simulink model "model_sim"  (R2016a)
settings: Solver=ode4  StartTime=0.0  StopTime=10.0  FixedStep=0.001  MaxStep=0.01  RelTol=1e-3
values from neighbouring files (symbols this model uses):
  lin = 1    [obiekt2.m]    (also in torque_x0.m; zad1.m = 10)
  p = 60    [zad1.m]
  Rn = 0.0185    [obiekt2.m]    (also in zad1.m)
libraries: simulink x2
settings Model: Creator=Maciek  LastModifiedBy=Maciek

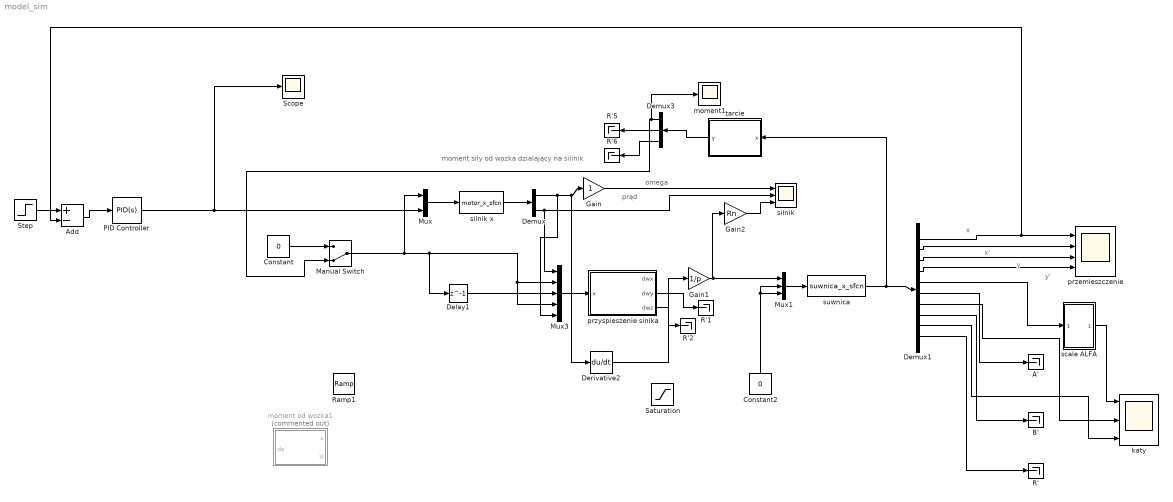
== system model_sim ==
  note: moment siły od wozka dzialający na silinik
  note: prąd
  note: omega
  note: y'
  note: y
  note: x'
  note: x
  A' : Terminator
  Add : Sum  Inputs=+-
  B' : Terminator
  Constant : Constant  Value=0
  Constant2 : Constant  Value=0
  Delay1 : Delay  DelayLength=1
  Demux : Demux  Outputs=2
  Demux1 : Demux  Outputs=10
  Demux3 : Demux  Outputs=3
  Derivative2 : Derivative
  Gain : Gain
  Gain1 : Gain  Gain=1/p
  Gain2 : Gain  Gain=Rn
  Manual Switch : ManualSwitch  CurrentSetting=0
  Mux : Mux  Inputs=2
  Mux1 : Mux  Inputs=3
  Mux3 : Mux  Inputs=5
  PID Controller : simulink/Continuous/PID Controller  Controller=PID  TimeDomain=Continuous-time  SampleTime=-1  IntegratorMethod=Forward Euler  FilterMethod=Forward Euler  Form=Parallel  UseFilter=on  ControllerParametersSource=internal  P=100  I=0.02  D=5  N=100  InitialConditionSource=internal  InitialConditionForIntegrator=0  InitialConditionForFilter=0  ExternalReset=none  LimitOutput=on  UpperSaturationLimit=20  LowerSaturationLimit=-20  LinearizeAsGain=on  AntiWindupMode=none  Kb=1  TrackingMode=off  Kt=1  PParamMin=[]  PParamMax=[]  IParamMin=[]  IParamMax=[]  DParamMin=[]  DParamMax=[]  NParamMin=[]  NParamMax=[]  KbParamMin=[]  KbParamMax=[]  KtParamMin=[]  KtParamMax=[]  POutMin=[]  POutMax=[]  IOutMin=[]  IOutMax=[]  DOutMin=[]  DOutMax=[]  NOutMin=[]  NOutMax=[]  KbOutMin=[]  KbOutMax=[]  KtOutMin=[]  KtOutMax=[]  IntegratorOutMin=[]  IntegratorOutMax=[]  FilterOutMin=[]  FilterOutMax=[]  SumOutMin=[]  SumOutMax=[]  SumI1OutMin=[]  SumI1OutMax=[]  SumI2OutMin=[]  SumI2OutMax=[]  SumI3OutMin=[]  SumI3OutMax=[]  SumDOutMin=[]  SumDOutMax=[]  SaturationOutMin=[]  SaturationOutMax=[]  IntegratorContinuousStateAttributes=''  IntegratorStateMustResolveToSignalObject=off  IntegratorRTWStateStorageClass=Auto  FilterContinuousStateAttributes=''  FilterStateMustResolveToSignalObject=off  FilterRTWStateStorageClass=Auto  DifferentiatorICPrevScaledInput=0  DifferentiatorOutMin=[]  DifferentiatorOutMax=[]
  R'{,1..2,5..6} (5 alike) : Terminator
  Ramp1 : simulink/Sources/Ramp  slope=0.5  start=0  X0=0
  Saturation : Saturate  UpperLimit=10  LowerLimit=-10
  Scope : Scope
  Step : Step  After=0.2  SampleTime=0
  katy : Scope  NumInputPorts=3
  moment od wozka1 : MATLAB Function  Commented=on  TreatAsAtomicUnit=on
  moment1 : Scope
  przemieszczenie : Scope  NumInputPorts=4
  przyspieszenie sinika : MATLAB Function  TreatAsAtomicUnit=on
  scale ALFA : Subsystem
  silnik : Scope  NumInputPorts=3
  silnik x : S-Function  FunctionName=motor_x_sfcn  SFunctionDeploymentMode=off  EnableBusSupport=off
  suwnica : S-Function  FunctionName=suwnica_x_sfcn  Parameters=x0  SFunctionDeploymentMode=off  EnableBusSupport=off
  tarcie : MATLAB Function  TreatAsAtomicUnit=on
  wires:
  Mux/1 -> silnik x/1
  silnik x/1 -> Demux/1
  Demux/1 -> Mux3/5, Derivative2/1, Gain/1
  Mux1/1 -> suwnica/1
  Constant2/1 -> Mux1/2, Mux1/3
  Demux1/10 -> R'/1
  Demux1/8 -> B'/1
  Demux1/7 -> katy/2
  Demux1/9 -> katy/3
  Demux1/6 -> A'/1
  Demux1/2 -> przemieszczenie/2
  Demux1/3 -> przemieszczenie/3
  Demux1/4 -> przemieszczenie/4
  Mux3/1 -> przyspieszenie sinika/1(x)
  przyspieszenie sinika/3(dwz) -> R'2/1
  przyspieszenie sinika/2(dwy) -> R'1/1
  suwnica/1 -> tarcie/1(x), Demux1/1
  Gain/1 -> silnik/1
  Demux/2 -> Mux3/1, silnik/2
  Delay1/1 -> Mux3/3
  Constant/1 -> Manual Switch/1
  Gain2/1 -> silnik/3
  tarcie/1(y) -> Demux3/1
  Demux3/2 -> R'5/1
  Demux3/3 -> R'6/1
  Demux3/1 -> moment1/1, Manual Switch/2
  Gain1/1 -> Mux1/1, Gain2/1
  Demux1/5 -> scale ALFA/1(In1)
  Demux1/1 -> Add/2, przemieszczenie/1
  scale ALFA/1(Out1) -> katy/1
  Manual Switch/1 -> Mux/1, Mux3/4, Mux3/2, Delay1/1
  PID Controller/1 -> Scope/1, Mux/2
  Add/1 -> PID Controller/1
  Step/1 -> Add/1
  Derivative2/1 -> Gain1/1

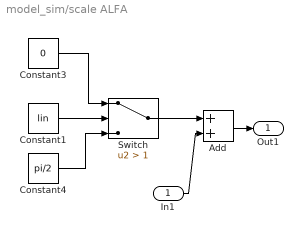
== system model_sim/scale ALFA ==
  In1 : Inport
  Add : Sum  Inputs=2
  Constant1 : Constant  Value=lin
  Constant3 : Constant  Value=0
  Constant4 : Constant  Value=pi/2
  Switch : Switch  Criteria=u2 > Threshold  Threshold=1
  Out1 : Outport
  wires:
  Add/1 -> Out1/1
  In1/1 -> Add/2
  Constant4/1 -> Switch/3
  Constant3/1 -> Switch/1
  Switch/1 -> Add/1
  Constant1/1 -> Switch/2

== matlab function model_sim/przyspieszenie sinika ==
  data: x input; dwx output; dwy output; dwz output
function [dwx, dwy, dwz] = angular_accel(x)

    %w = x(1); %predkosc katowa
    %temp = x(1);
    %ix = temp(2);
    wx = x(5);
    ix = x(1); % prad x
    iy = x(2); % prad x
    awx = x(3); %przysp x
    awy = x(4); %przys y
    
    xs = 1.5;   % szerokość suwnicy
    sy = 2.5;   % dł suwnicy
    mw = 1.155;%2.49;  % masa wózka
    ms = 2.2;%4.09;  % masa szyny
    mc = 1;     % masa ciężarka
    Rn = 0.0185;% promien bloków napedzajacych
    g = 9.81;
    p = 60;%przekladnia
    
    J = 1.1418*10^(-6);   %moment bezwladnisci
    tau_e = 0.48*10^(-3);
    tau_m = 21*10^(-3);                                                                             
    Ke = 0.02607;  %stala elektryczna
    Km = 0.0265;    %stala mechaniczna
    R = 12.5;      %opornosc
    L = 5.93*10^(-3);    %indukcyjnosc
    
    Mx = mw + mc;
    My = mw + ms + mc;
    
    dwx = (Km * ix - awx * Mx * Rn /p - 0* wx) / J;
    
    dwy = (Km * iy - awy * My * Rn / p ) / J;
    
    dwz = 0;%Km/J * i - aw * Mx * Rn / J;
    
end

== matlab function model_sim/tarcie ==
  data: x input; y output
function y  = tarcie(x)
%#codegen

    xs = 1.5;   % szerokość suwnicy
    sy = 2.5;   % dł suwnicy
    mw = 1.155;%2.49;  % masa wózka
    ms = 2.2;%4.09;  % masa szyny
    mc = 1;     % masa ciężarka
    Rn = 0.0185;% promien bloków napedzajacych
    g = 9.81;
    
    k1 = 82;%75;
    k2 = 100;%75;
    k3 = 75;%75;
    %siły tarcia
    if x(2) > 0 
        Tx = k1*mw*x(2) + 7.5;%10;
    elseif x(2) < 0
        Tx = k1*mw*x(2) - 7.5;%10;
    else
        Tx = 0;
    end
    if x(4) > 0 
        Ty = k2*(mw+ms)*x(4) + 5;%22;
    elseif x(4) < 0
        Ty = k2*(mw+ms)*x(4) - 5;%22;
    else
        Ty = 0;
    end
    if x(10) > 0
        Tr = -g*mc - x(10) * k3;%142;
    elseif x(10) < 0 
        Tr = g*mc - x(10) * k3;%218;
    else
        Tr = g*mc;
    end
    %Tr = k3*mc*x(10);
    
    T1 = Tx/mw;
    T2 = Ty/(mw+mc);
    T3 = Tr/mc;
    y = zeros(3,1);
    y(1) = T1;
    y(2) = T2;
    y(3) = T3;
end

== matlab function model_sim/moment od wozka1 ==
  data: x input; dx output; U input
function dx   = torque_x(x, U)

    lin = 1;
    xs = 1.5;   % szerokość suwnicy
    sy = 2.5;   % dł suwnicy
    mw = 1.155;%2.49;  % masa wózka
    ms = 2.2;%4.09;  % masa szyny
    mc = 1;     % masa ciężarka
    Rn = 0.0185;% promien bloków napedzajacych
    g = 9.81;
    
    %wsp tarcia
    k1 = 82;%75;
    k2 = 100;%75;
    k3 = 75;%75;
    %siły tarcia
    if x(2) > 0 
        Tx = k1*mw*x(2) + 7.5;%10;
    elseif x(2) < 0
        Tx = k1*mw*x(2) - 7.5;%10;
    else
        Tx = 0;
    end
    if x(4) > 0 
        Ty = k2*(mw+ms)*x(4) + 5;%22;
    elseif x(4) < 0
        Ty = k2*(mw+ms)*x(4) - 5;%22;
    else
        Ty = 0;
    end
    if x(10) > 0
        Tr = -g*mc - x(10) * k3;%142;
    elseif x(10) < 0 
        Tr = g*mc - x(10) * k3;%218;
    else
        Tr = 0;
    end
    %Tr = k3*mc*x(10);
    
    T1 = Tx/mw;
    T2 = Ty/(mw+mc);
    T3 = Tr/mc;
    
    %u = [x(11) x(12) x(13)];
    u = U * Rn; % przejscie z przyspieszenia katowego na liniowe
    N1 = u(1) - T1;
    N2 = u(2) - T2;
    N3 = u(3) - T3;
    
    ni1 = mc/mw;
    ni2 = mc/(mw + ms);
    
    if lin == 1%model liniowy
        dx= zeros(3,1);
        dx(1) = N1-ni1*x(5)*N3;                             %xw'
        dx(2) = N2+ni2*x(7)*N3;                             %yw'
        dx(3) = -N3 +g;                                    %R'
    
    else %model nieliniowy
        dx= zeros(3,1);
        
        V5 = cos(x(5))*sin(x(5))*(x(8))^2*x(9) - 2*x(10)*x(6) + g*cos(x(5))*cos(x(7));
        V6 = 2*x(8)*(cos(x(5))*x(6)*x(9) + sin(x(5))*x(10)) + g*sin(x(7));
        V7 = (sin(x(5)))^2*(x(8))^2*x(9) + g*sin(x(5))*cos(x(7)) + x(6)*x(6)*x(9);
        
        dx(1) = N1+ni1*cos(x(5))*N3;
        dx(2) = N2 + ni2*sin(x(7))*sin(x(5))*N3;
        dx(3) = -cos(x(5))*N1 - sin(x(5))*sin(x(7))*N2 -(1+ni1*(cos(x(5)))^2+ni2*(sin(x(5)))^2*(sin(x(7)))^2)*N3+V7;
     end
    
end
